simulink library "csu_fec_filter_error_check_lib"  (R2014b)
settings: Solver=ode45  SolverMode=SingleTasking  StartTime=0.0  StopTime=10.0  RelTol=1e-3
undefined symbols (not defined in the file or in its folder): fcv_numerical_fault, fec_eps, kfl_n_state
libraries: simulink x3, util_info_lib x1
settings Model: Creator=escrane  LastModifiedBy=mstewart

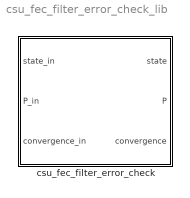
== system csu_fec_filter_error_check_lib ==
  csu_fec_filter_error_check : Subsystem

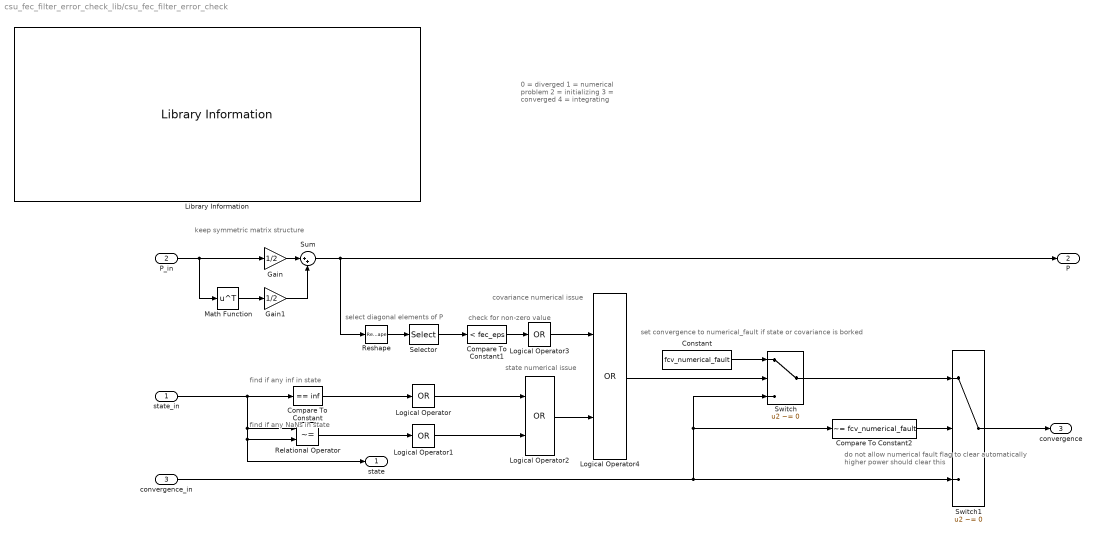
== system csu_fec_filter_error_check_lib/csu_fec_filter_error_check ==
  note: do not allow numerical fault flag to clear automatically
      | higher power should clear this
  note: set convergence to numerical_fault if state or covariance is borked
  note: covariance numerical issue
  note: state numerical issue
  note: check for non-zero value
  note: select diagonal elements of P
  note: find if any inf in state
  note: keep symmetric matrix structure
  note: 0 = diverged
      | 1 = numerical problem
      | 2 = initializing
      | 3 = converged
      | 4 = integrating
  note: find if any NaNs in state
  state_in : Inport
  P_in : Inport  Port=2
  convergence_in : Inport  Port=3
  Compare To Constant : simulink/Logic and Bit Operations/Compare To Constant  relop===  const=inf  OutDataTypeStr=boolean
  Compare To Constant1 : simulink/Logic and Bit Operations/Compare To Constant  relop=<  const=fec_eps  OutDataTypeStr=boolean
  Compare To Constant2 : simulink/Logic and Bit Operations/Compare To Constant  relop=~=  const=fcv_numerical_fault  OutDataTypeStr=boolean
  Constant : Constant  Value=fcv_numerical_fault  OutDataTypeStr=double
  Gain : Gain  Gain=1/2  OutDataTypeStr=double
  Gain1 : Gain  Gain=1/2  OutDataTypeStr=double
  Library Information : util_info_lib/Library Information  owner='escrane'
  Logical Operator : Logic  Operator=OR  Inputs=1  AllPortsSameDT=off  OutDataTypeStr=boolean
  Logical Operator1 : Logic  Operator=OR  Inputs=1  AllPortsSameDT=off  OutDataTypeStr=boolean
  Logical Operator2 : Logic  Operator=OR  AllPortsSameDT=off  OutDataTypeStr=boolean
  Logical Operator3 : Logic  Operator=OR  Inputs=1  AllPortsSameDT=off  OutDataTypeStr=boolean
  Logical Operator4 : Logic  Operator=OR  AllPortsSameDT=off  OutDataTypeStr=boolean
  Math Function : Math  Operator=transpose  OutputSignalType=real  SaturateOnIntegerOverflow=on
  Relational Operator : RelationalOperator  Operator=~=  OutDataTypeStr=boolean
  Reshape : Reshape
  Selector : Selector  InputPortWidth=fcv_n_elements  Indices=fcv_diag_elements
  Sum : Sum  Inputs=|++
  Switch : Switch  Criteria=u2 ~= 0
  Switch1 : Switch  Criteria=u2 ~= 0
  state : Outport  InitialOutput=zeros(kfl_n_state,1)
  P : Outport  Port=2  InitialOutput=zeros(kfl_n_state, kfl_n_state)
  convergence : Outport  Port=3  InitialOutput=zeros(kfl_n_state, kfl_n_state)
  wires:
  P_in/1 -> Math Function/1, Gain/1
  Math Function/1 -> Gain1/1
  Gain/1 -> Sum/1
  Gain1/1 -> Sum/2
  state_in/1 -> state/1, Relational Operator/2, Relational Operator/1, Compare To Constant/1
  Compare To Constant/1 -> Logical Operator/1
  Relational Operator/1 -> Logical Operator1/1
  Logical Operator/1 -> Logical Operator2/1
  Logical Operator1/1 -> Logical Operator2/2
  Reshape/1 -> Selector/1
  Sum/1 -> Reshape/1, P/1
  Selector/1 -> Compare To Constant1/1
  Compare To Constant1/1 -> Logical Operator3/1
  Logical Operator3/1 -> Logical Operator4/1
  Logical Operator2/1 -> Logical Operator4/2
  Constant/1 -> Switch/1
  Logical Operator4/1 -> Switch/2
  convergence_in/1 -> Switch1/3, Switch/3, Compare To Constant2/1
  Compare To Constant2/1 -> Switch1/2
  Switch1/1 -> convergence/1
  Switch/1 -> Switch1/1
